simulink model "Load_FFW_5Hz_PD"  (R2025a)
settings: Solver=VariableStepAuto  StartTime=0.0  StopTime=10.0  RelTol=1e-3
settings Model: Creator=Bramv  LastModifiedBy=Bramv

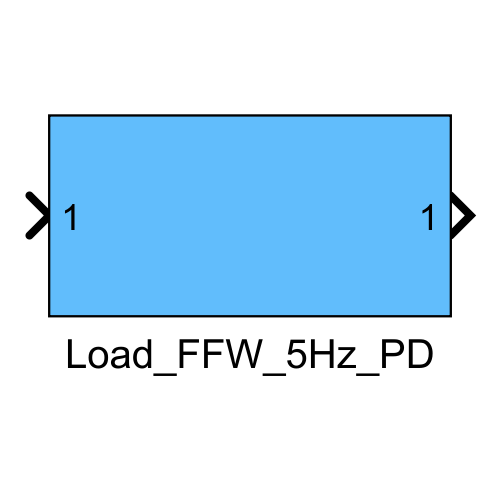
[thumbnail: Simulink's stored preview of the top-level diagram]
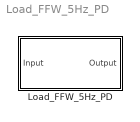
== system Load_FFW_5Hz_PD ==
  Load_FFW_5Hz_PD : Subsystem

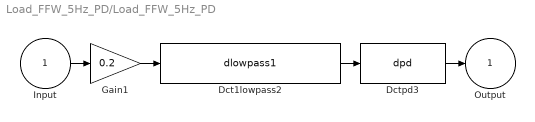
== system Load_FFW_5Hz_PD/Load_FFW_5Hz_PD ==
  Input : Inport
  Dct1lowpass2 : S-Function  FunctionName=dlowpass1  Parameters=f_den, 0.001  SFunctionDeploymentMode=off  EnableBusSupport=off  mask(dctools){f_den=20}
      mask prompts: f_den "Pole [Hz]"
      mask help: This block implements a discrete time 1st order lowpass filter.
      mask Display: disp('DCT 1st order lowpass')
  Dctpd3 : S-Function  FunctionName=dpd  Parameters=kp, kv, 0.001  SFunctionDeploymentMode=off  EnableBusSupport=off  mask(dctools){kp=1, kv=0.031831}
      mask help: This block implements a discrete time pd filter.
      mask Display: disp('DCT pd')
  Gain1 : Gain  Gain=0.2
  Output : Outport
  wires:
  Input/1 -> Gain1/1
  Gain1/1 -> Dct1lowpass2/1
  Dct1lowpass2/1 -> Dctpd3/1
  Dctpd3/1 -> Output/1
